simulink subsystem "accurateTiltingModel"  (R2022b)
settings: Solver=VariableStepAuto  StartTime=0.0  StopTime=10.0  RelTol=1e-3
undefined symbols (not defined in the file): Angle, Axis, I_b, I_i, k_m
libraries: matrix_library x2, robotcorelib x2, sharedutil x1
settings Model: Creator=pozzan  LastModifiedBy=pozzan

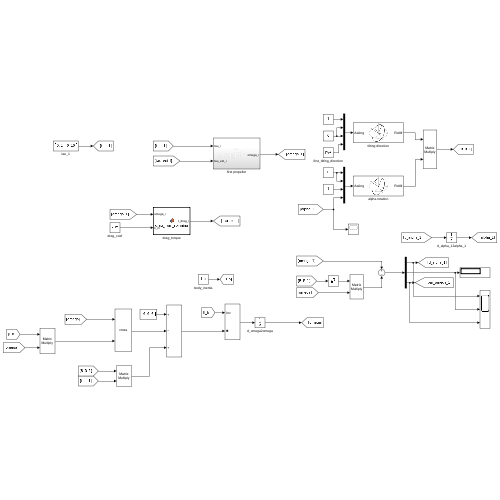
[thumbnail: Simulink's stored preview of the top-level diagram]
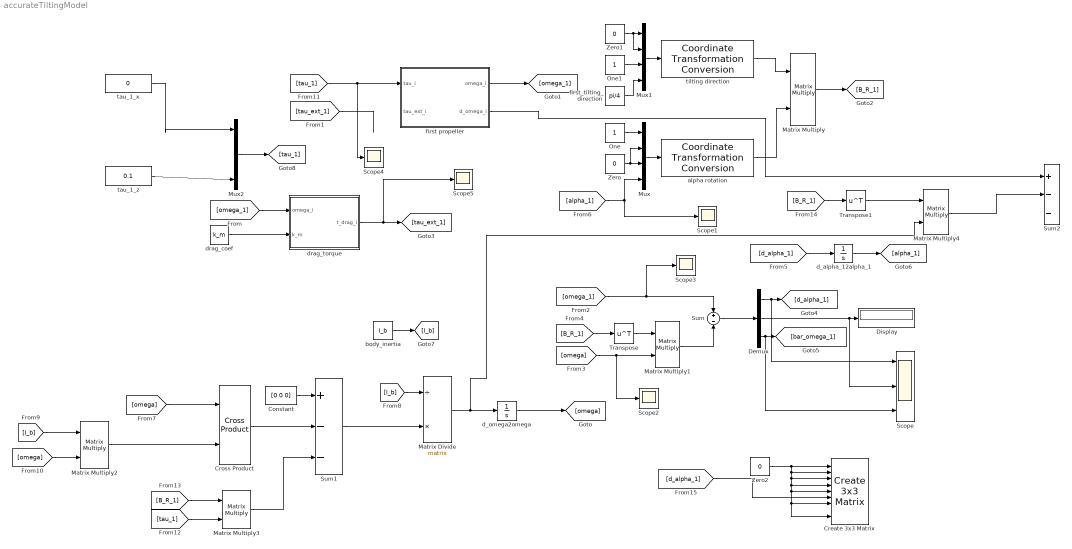
== system accurateTiltingModel ==
  Constant : Constant  Value=[0 0 0]
  Create 3x3 Matrix : sharedutil/Create 3x3 Matrix  aMode=aMode
      settings: LibrarySourceBlock=aerolibutil/Create 3x3 Matrix
  Cross Product : matrix_library/Cross Product
  Demux : Demux  Outputs=3
  Display : Display
  Matrix Divide : Product  Inputs=/*  Multiplication=Matrix(*)
  Matrix Multiply{,1..4} (5 alike) : Product  Multiplication=Matrix(*)
  Mux : Mux
  Mux1 : Mux
  Mux2 : Mux  Inputs=3
  One : Constant  OutDataTypeStr=Inherit: Inherit via back propagation
  One1 : Constant  OutDataTypeStr=Inherit: Inherit via back propagation
  Scope : Scope  NumInputPorts=3
  Scope{1..5} (5 alike) : Scope
  Sum : Sum  Inputs=+-
  Sum1 : Sum  Inputs=+--
  Sum2 : Sum  Inputs=+--
  Transpose : Math  Operator=transpose
  Transpose1 : Math  Operator=transpose
  Zero : Constant  Value=0  OutDataTypeStr=Inherit: Inherit via back propagation
  Zero1 : Constant  Value=0  OutDataTypeStr=Inherit: Inherit via back propagation
  Zero2 : Constant  Value=0  OutDataTypeStr=Inherit: Inherit via back propagation
  alpha rotation : robotcorelib/Coordinate Transformation Conversion  InputRepresentation=Axis-Angle  InputEulerSequence=ZYX  ShowTrVecInputPort=on  OutputRepresentation=Rotation Matrix  OutputEulerSequence=ZYX  ShowTrVecOutputPort=on  SimulateUsing=Code generation
  body_inertia : Constant  Value=I_b
  d_alpha_12alpha_1 : Integrator  InitialCondition=0.1
  d_omega2omega : Integrator  InitialCondition=[0 0 0]
  drag_coef : Constant  Value=k_m
  drag_torque : MATLAB Function  TreatAsAtomicUnit=on
  first propeller : Subsystem
  first_tilting_direction : Constant  Value=pi/4
  tau_1_x : Constant  Value=0
  tau_1_z : Constant  Value=0.1
  tilting direction : robotcorelib/Coordinate Transformation Conversion  InputRepresentation=Axis-Angle  InputEulerSequence=ZYX  ShowTrVecInputPort=on  OutputRepresentation=Rotation Matrix  OutputEulerSequence=ZYX  ShowTrVecOutputPort=on  SimulateUsing=Code generation
  wires:
  drag_coef/1 -> drag_torque/2(k_m)
  [tau_1] -> first propeller/1(tau_i), Scope4/1
  [tau_ext_1] -> ?
  first propeller/1(omega_i) -> [omega_1]
  d_omega2omega/1 -> [omega]
  alpha rotation/1 -> Matrix Multiply/2
  tilting direction/1 -> Matrix Multiply/1
  Matrix Multiply/1 -> [B_R_1]
  Mux/1 -> alpha rotation/1
  Zero/1 -> Mux/3, Mux/2
  One/1 -> Mux/1
  One1/1 -> Mux1/3
  Zero1/1 -> Mux1/2, Mux1/1
  Mux1/1 -> tilting direction/1
  first_tilting_direction/1 -> Mux1/4
  [omega_1] -> drag_torque/1(omega_i)
  drag_torque/1(t_drag_i) -> [tau_ext_1], Scope5/1
  [omega_1] -> Sum/1, Scope3/1
  [B_R_1] -> Transpose/1
  Transpose/1 -> Matrix Multiply1/1
  [omega] -> Scope2/1, Matrix Multiply1/2
  Matrix Multiply1/1 -> Sum/2
  Sum/1 -> Demux/1
  Demux/1 -> [d_alpha_1], Scope/1
  Demux/2 -> Display/1, Scope/2
  Demux/3 -> [bar_omega_1], Scope/3
  [d_alpha_1] -> d_alpha_12alpha_1/1
  d_alpha_12alpha_1/1 -> [alpha_1]
  [alpha_1] -> Mux/4, Scope1/1
  Matrix Divide/1 -> d_omega2omega/1, Matrix Multiply4/2
  body_inertia/1 -> [I_b]
  [omega] -> Cross Product/1
  Matrix Multiply2/1 -> Cross Product/2
  [I_b] -> Matrix Multiply2/1
  Cross Product/1 -> Sum1/2
  [omega] -> Matrix Multiply2/2
  Matrix Multiply3/1 -> Sum1/3
  Constant/1 -> Sum1/1
  [I_b] -> Matrix Divide/1
  Sum1/1 -> Matrix Divide/2
  tau_1_x/1 -> Mux2/1
  [tau_1] -> Matrix Multiply3/2
  [B_R_1] -> Matrix Multiply3/1
  Mux2/1 -> [tau_1]
  tau_1_z/1 -> Mux2/3
  first propeller/2(d_omega_i) -> Sum2/1
  Matrix Multiply4/1 -> Sum2/2
  Transpose1/1 -> Matrix Multiply4/1
  [B_R_1] -> Transpose1/1
  Zero2/1 -> Create 3x3 Matrix/1, Create 3x3 Matrix/2, Create 3x3 Matrix/3, Create 3x3 Matrix/4, Create 3x3 Matrix/5, Create 3x3 Matrix/9, Create 3x3 Matrix/7
  [d_alpha_1] -> Create 3x3 Matrix/6

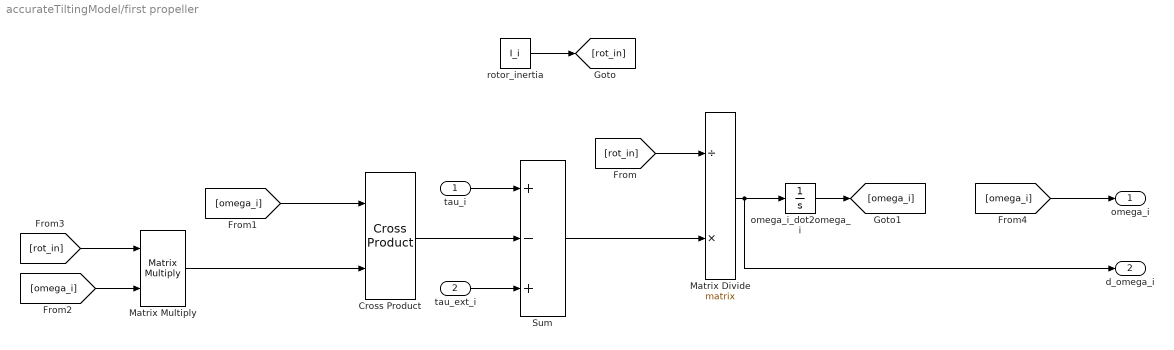
== system accurateTiltingModel/first propeller ==
  tau_i : Inport  PortDimensions=3
  tau_ext_i : Inport  Port=2  PortDimensions=3
  Cross Product : matrix_library/Cross Product
  Matrix Divide : Product  Inputs=/*  Multiplication=Matrix(*)
  Matrix Multiply : Product  Multiplication=Matrix(*)
  Sum : Sum  Inputs=+-+
  omega_i_dot2omega_i : Integrator  InitialCondition=[0 0 0]
  rotor_inertia : Constant  Value=I_i
  omega_i : Outport
  d_omega_i : Outport  Port=2
  wires:
  tau_i/1 -> Sum/1
  Sum/1 -> Matrix Divide/2
  [omega_i] -> Matrix Multiply/2
  [rot_in] -> Matrix Multiply/1
  Matrix Multiply/1 -> Cross Product/2
  Cross Product/1 -> Sum/2
  [omega_i] -> Cross Product/1
  tau_ext_i/1 -> Sum/3
  [omega_i] -> omega_i/1
  rotor_inertia/1 -> [rot_in]
  omega_i_dot2omega_i/1 -> [omega_i]
  Matrix Divide/1 -> d_omega_i/1, omega_i_dot2omega_i/1
  [rot_in] -> Matrix Divide/1

== matlab function accurateTiltingModel/drag_torque ==
  data: omega_i input; k_m input; t_drag_i output
function t_drag_i = drag_from_spinning(omega_i, k_m)

t_drag_i = [0; 0; -k_m*omega_i(3)*abs(omega_i(3))];
